simulink model "final"  (R2021a)
settings: Solver=FixedStepDiscrete  StartTime=0.0  StopTime=inf  FixedStep=0.05  RelTol=1e-3  EnableMultiTasking=on
undefined symbols (not defined in the file): c, Sat
libraries: arduinolib x6, pid_lib x1, arduinosensorlib x1
settings Model: SimulationMode=external  SILPILModeSetting=veronly  ExtModeEnableFloating=off  ExtModeTrigDuration=1  Creator=alire  LastModifiedBy=alire
settings OptimizationCC: EnhancedBackFolding=on  PassReuseOutputArgsThreshold=0  MaxStackSize=64  OptimizeBlockOrder=speed  DifferentSizesBufferReuse=on  OptimizationCustomize=off
settings DebuggingCC: ParameterTunabilityLossMsg=error
settings HardwareCC: ProdBitPerInt=16  ProdBitPerPointer=16  ProdBitPerSizeT=16  ProdBitPerPtrDiffT=16  ProdLargestAtomicFloat=None  ProdWordSize=8  ProdHWDeviceType=Atmel->AVR  UseEmbeddedCoderFeatures=off
settings SFSimCC: MATLABDynamicMemAlloc=off
settings RTWCC: SystemTargetFile=ert.tlc  HardwareBoard=Arduino Uno  TemplateMakefile=ert_default_tmf  Toolchain=Arduino AVR  BuildConfiguration=Faster Runs
settings CodeAppCC: ForceParamTrailComments=on  OperatorAnnotations=on
settings ERTTargetCC: ERTCustomFileBanners=off  SupportContinuousTime=on  SupportNonInlinedSFcns=on  RemoveResetFunc=off  SupportVariableSizeSignals=on  ModelStepFunctionPrototypeControlCompliant=off  ExtMode=on  ExtModeStaticAllocSize=250  ExtModeMexArgs='127.0.0.1' 0 17725  ERTSrcFileBannerTemplate=codertarget_code_template.cgt  ERTHdrFileBannerTemplate=codertarget_code_template.cgt  ERTDataSrcFileTemplate=codertarget_code_template.cgt  ERTDataHdrFileTemplate=codertarget_code_template.cgt

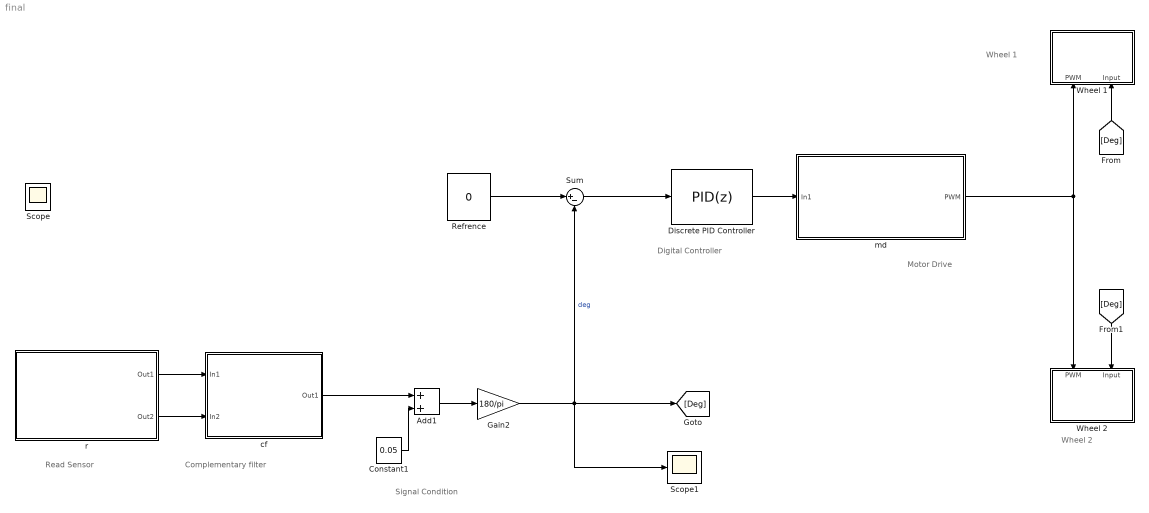
== system final ==
  note: Read Sensor
  note: Complementary filter
  note: Signal Condition
  note: Motor Drive
  note: Wheel 1
  note: Wheel 2
  note: Digital Controller
  Add1 : Sum
  Constant1 : Constant  Value=0.05  SampleTime=-1
  Discrete PID Controller : pid_lib/PID Controller  Controller=PID  Form=Parallel  TimeDomain=Discrete-time  UseExternalTs=off  SampleTime=-1  IntegratorMethod=Forward Euler  FilterMethod=Forward Euler  ControllerParametersSource=internal  P=30  I=0  D=4  UseFilter=off  N=100  TunerSelectOption=Transfer Function Based (PID Tuner App)  InitialConditionSource=internal  InitialConditionForIntegrator=0  InitialConditionForFilter=0  DifferentiatorICPrevScaledInput=0  ExternalReset=none  TrackingMode=off  Kt=1  LimitOutput=off  SatLimitsSource=internal  UpperSaturationLimit=inf  LowerSaturationLimit=-inf  LinearizeAsGain=off  AntiWindupMode=none  Kb=1  POutMin=[]  POutMax=[]  IOutMin=[]  IOutMax=[]  DOutMin=[]  DOutMax=[]  NOutMin=[]  NOutMax=[]  SumOutMin=[]  SumOutMax=[]  SaturationOutMin=[]  SaturationOutMax=[]  PParamMin=[]  PParamMax=[]  IParamMin=[]  IParamMax=[]  DParamMin=[]  DParamMax=[]  NParamMin=[]  NParamMax=[]  KbParamMin=[]  KbParamMax=[]  KtParamMin=[]  KtParamMax=[]  KbOutMin=[]  KbOutMax=[]  KtOutMin=[]  KtOutMax=[]  IntegratorOutMin=[]  IntegratorOutMax=[]  FilterOutMin=[]  FilterOutMax=[]  SumI1OutMin=[]  SumI1OutMax=[]  SumI2OutMin=[]  SumI2OutMax=[]  SumI3OutMin=[]  SumI3OutMax=[]  SumI4OutMin=[]  SumI4OutMax=[]  SumDOutMin=[]  SumDOutMax=[]  DifferentiatorOutMin=[]  DifferentiatorOutMax=[]  FilterDiffOutCoefMin=[]  FilterDiffOutCoefMax=[]  ReciprocalOutMin=[]  ReciprocalOutMax=[]  SumDenOutMin=[]  SumDenOutMax=[]  SumNumOutMin=[]  SumNumOutMax=[]  DivideOutMin=[]  DivideOutMax=[]  UdiffTsProdOutMin=[]  UdiffTsProdOutMax=[]  NTsProdOutMin=[]  NTsProdOutMax=[]  UintegralTsProdOutMin=[]  UintegralTsProdOutMax=[]  UngainTsProdOutMin=[]  UngainTsProdOutMax=[]  IntegratorContinuousStateAttributes=''  IntegratorStateMustResolveToSignalObject=off  IntegratorRTWStateStorageClass=Auto  FilterContinuousStateAttributes=''  FilterStateMustResolveToSignalObject=off  FilterRTWStateStorageClass=Auto  ParallelPVariant=InternalParameters  IdealPVariant=Disabled  IVariant=InternalParameters  DVariant=InternalParameters  IntegratorVariant=Discrete  SatVariant=Disabled  AWVariant=Passthrough  PCopyVariant=Disabled  TRVariant=Disabled  FdbkBlocksVariant=Forward  IdealPFdbkVariant=Disabled  SatFdbkVariant=Disabled  DerivativeFilterVariant=Differentiator  NVariant=Passthrough  NCopyVariant=Disabled_SignalSpec  FilterICVariant=InternalICsDifferentiator  IntegratorICVariant=InternalICs  ExternalResetVariant=Disabled  TRSumVariant=Passthrough  SumFdbkVariant=Disabled  SumVariant=Sum_PID  TsampFilterVariant=InternalTs  TsampNgainVariant=Passthrough  TsampIntegralVariant=Passthrough  ExternalSaturationOutDataTypeStr=Inherit: Same as second input
  Gain2 : Gain  Gain=180/pi
  Refrence : Constant  Value=0  SampleTime=-1
  Scope1 : Scope
  Sum : Sum  Inputs=|+-
  Wheel 1 : Subsystem
  Wheel 2 : Subsystem
  cf : Subsystem
  md : Subsystem
  r : Subsystem
  Scope : Scope
  wires:
  Refrence/1 -> Sum/1
  r/1(Out1) -> cf/1(In1)
  r/2(Out2) -> cf/2(In2)
  Constant1/1 -> Add1/2
  Add1/1 -> Gain2/1
  cf/1(Out1) -> Add1/1
  Gain2/1 -> [Deg], Sum/2, Scope1/1  "deg"
  Discrete PID Controller/1 -> md/1(In1)
  md/1(PWM) -> Wheel 2/1(PWM), Wheel 1/1(PWM)
  [Deg] -> Wheel 1/2(Input)
  [Deg] -> Wheel 2/2(Input)
  Sum/1 -> Discrete PID Controller/1

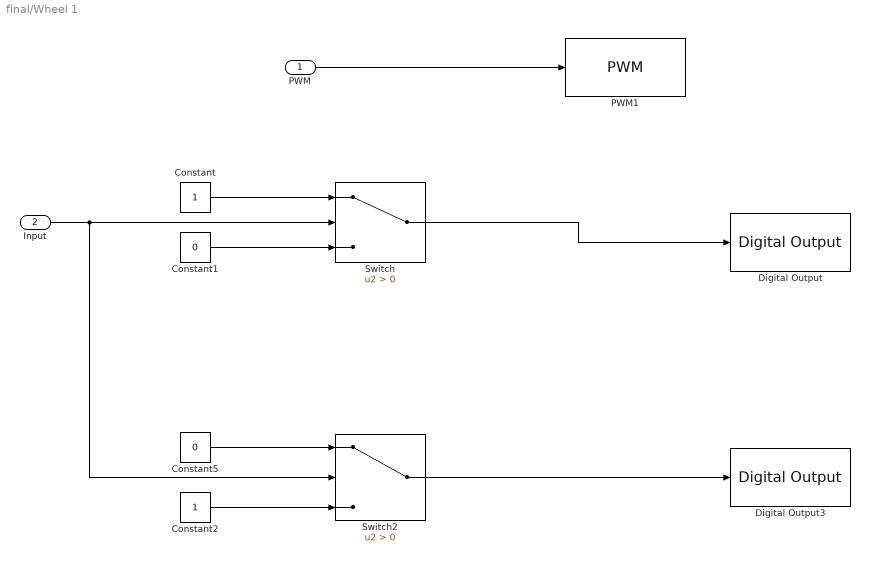
== system final/Wheel 1 ==
  PWM : Inport
  Input : Inport  Port=2
  Constant : Constant
  Constant1 : Constant  Value=0
  Constant2 : Constant
  Constant5 : Constant  Value=0
  Digital Output : arduinolib/Digital Output  pinNumber=6  Direction=output  blockPlatform=arduino
  Digital Output3 : arduinolib/Digital Output  pinNumber=7  Direction=output  blockPlatform=arduino
  PWM1 : arduinolib/PWM  pinNumber=5  frequencyType=Default  desiredFrequency=490.2  achievableFrequency=490.2
  Switch : Switch  Criteria=u2 > Threshold
  Switch2 : Switch  Criteria=u2 > Threshold
  wires:
  PWM/1 -> PWM1/1
  Input/1 -> Switch2/2, Switch/2
  Constant1/1 -> Switch/3
  Switch/1 -> Digital Output/1
  Constant/1 -> Switch/1
  Switch2/1 -> Digital Output3/1
  Constant5/1 -> Switch2/1
  Constant2/1 -> Switch2/3

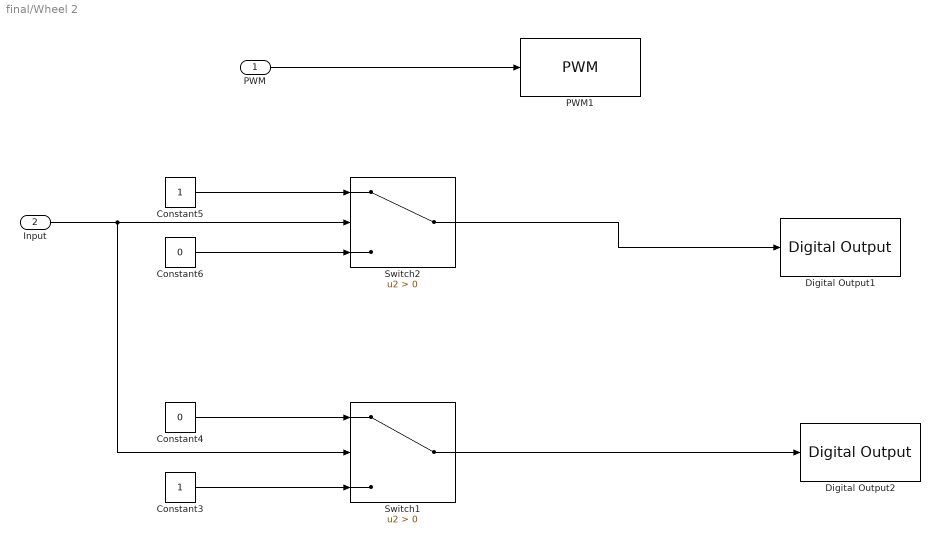
== system final/Wheel 2 ==
  PWM : Inport
  Input : Inport  Port=2
  Constant3 : Constant
  Constant4 : Constant  Value=0
  Constant5 : Constant
  Constant6 : Constant  Value=0
  Digital Output1 : arduinolib/Digital Output  pinNumber=8  Direction=output  blockPlatform=arduino
  Digital Output2 : arduinolib/Digital Output  pinNumber=9  Direction=output  blockPlatform=arduino
  PWM1 : arduinolib/PWM  pinNumber=10  frequencyType=Default  desiredFrequency=490.2  achievableFrequency=490.2
  Switch1 : Switch  Criteria=u2 > Threshold
  Switch2 : Switch  Criteria=u2 > Threshold
  wires:
  PWM/1 -> PWM1/1
  Input/1 -> Switch1/2, Switch2/2
  Constant5/1 -> Switch2/1
  Switch2/1 -> Digital Output1/1
  Constant6/1 -> Switch2/3
  Switch1/1 -> Digital Output2/1
  Constant3/1 -> Switch1/3
  Constant4/1 -> Switch1/1

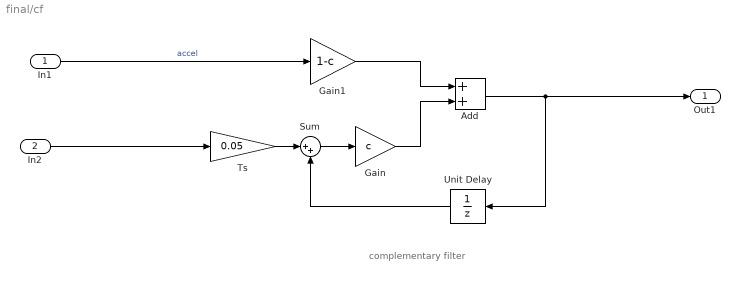
== system final/cf ==
  note: complementary filter
  In1 : Inport
  In2 : Inport  Port=2
  Add : Sum
  Gain : Gain  Gain=c
  Gain1 : Gain  Gain=1-c
  Sum : Sum  Inputs=|++
  Ts : Gain  Gain=0.05
  Unit Delay : UnitDelay  SampleTime=-1  HasFrameUpgradeWarning=on
  Out1 : Outport
  wires:
  In2/1 -> Ts/1
  Sum/1 -> Gain/1
  Ts/1 -> Sum/1
  Unit Delay/1 -> Sum/2
  In1/1 -> Gain1/1  "accel"
  Add/1 -> Out1/1, Unit Delay/1
  Gain/1 -> Add/2
  Gain1/1 -> Add/1

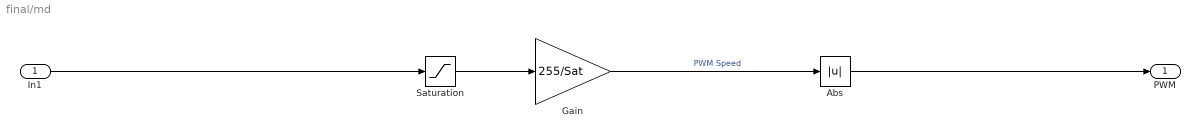
== system final/md ==
  In1 : Inport
  Abs : Abs
  Gain : Gain  Gain=255/Sat
  Saturation : Saturate  UpperLimit=Sat  LowerLimit=-Sat
  PWM : Outport
  wires:
  In1/1 -> Saturation/1
  Saturation/1 -> Gain/1
  Gain/1 -> Abs/1  "PWM Speed"
  Abs/1 -> PWM/1

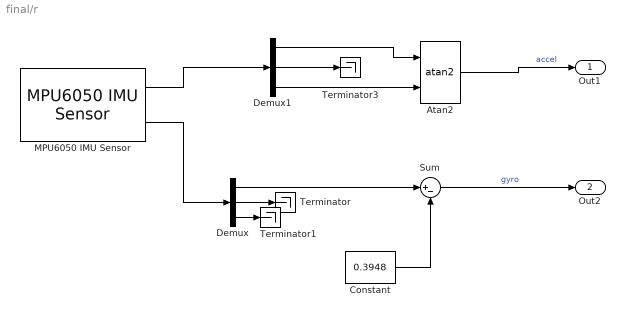
== system final/r ==
  Atan2 : Trigonometry  Operator=atan2
  Constant : Constant  Value=0.3948  SampleTime=-1
  Demux : Demux  Outputs=3
  Demux1 : Demux  Outputs=3
  MPU6050 IMU Sensor : arduinosensorlib/MPU6050 IMU Sensor  SlaveAddress=0x68  Accel=on  AngularRate=on  Temperature=off  Status=off  EulerAngles=off  Quat=off  AccelRange=2G  GyroRange=250 dps  DmpOdr=200 Hz  Dlpf=Accelerometer: 10Hz, Gyroscope: 10Hz  SampleTime=-1
      settings: SourceProductBaseCode=ARDUINO
  Sum : Sum  Inputs=|+-
  Terminator : Terminator
  Terminator1 : Terminator
  Terminator3 : Terminator
  Out1 : Outport
  Out2 : Outport  Port=2
  wires:
  Demux1/2 -> Terminator3/1
  MPU6050 IMU Sensor/1 -> Demux1/1
  Sum/1 -> Out2/1  "gyro"
  Demux/1 -> Sum/1
  Demux/3 -> Terminator1/1
  MPU6050 IMU Sensor/2 -> Demux/1
  Demux1/1 -> Atan2/1
  Demux/2 -> Terminator/1
  Constant/1 -> Sum/2
  Demux1/3 -> Atan2/2
  Atan2/1 -> Out1/1  "accel"
